simulink model "Simulink4"  (Simulink 5.0)
settings: Solver=ode45  StartTime=0.0  StopTime=100.0  RelTol=1e-5
libraries: simulink x1
settings Model: LastModifiedBy=stevel

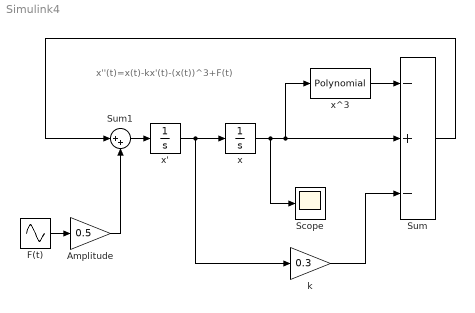
== system Simulink4 ==
  note: x''(t)=x(t)-kx'(t)-(x(t))^3+F(t)
  Amplitude : Gain  Gain=0.5  SaturateOnIntegerOverflow=on
  F(t) : Sin  Frequency=1.25  Phase=pi/2  SampleTime=0
  Scope : Scope
  Sum : Sum  Inputs=-+-  SaturateOnIntegerOverflow=on
  Sum1 : Sum  Inputs=|++  SaturateOnIntegerOverflow=on
  k : Gain  Gain=0.3  SaturateOnIntegerOverflow=on
  x : Integrator  InitialCondition=1
  x' : Integrator  InitialCondition=1
  x^3 : simulink/Math Operations/Polynomial  coefs=[1,0,0,0]
  wires:
  x'/1 -> x/1, k/1
  x/1 -> Scope/1, Sum/2, x^3/1
  Sum1/1 -> x'/1
  k/1 -> Sum/3
  Sum/1 -> Sum1/1
  x^3/1 -> Sum/1
  F(t)/1 -> Amplitude/1
  Amplitude/1 -> Sum1/2
